simulink model "T_TypeInvPOb_07042020"  (R2018a)
settings: Solver=VariableStepDiscrete  StartTime=0.0  StopTime=0.4  MaxStep=1e-4  RelTol=1e-3  EnableMultiTasking=on
InitFcn:
  | Fs=10000;
  | Ts = 1/Fs; Vd = 400;
  | Vrate = 220; Irate = 25;
  | Rload = Vrate/Irate;
  | 
  | 
  | Lf = 0.423e-3+0.429e-3; Cf = 20e-6;
  | Rf = 0.01; Rc = 0.05;
  | 
  | C = 470e-6;
libraries: powerlib x28, powerlib_meascontrol x1
settings Model: Creator=Nguyen Linh  LastModifiedBy=ADMIN
settings SolverCC: ZeroCrossAlgorithm=Adaptive  AutoInsertRateTranBlk=on
settings DataIOCC: LimitDataPoints=on  SaveFormat=Array
settings OptimizationCC: LifeSpan=inf
settings DebuggingCC: MaxConsecutiveZCsMsg=none  SFUnexpectedBacktrackingDiag=warning  SFNoUnconditionalDefaultTransitionDiag=warning  SFExecutionAtInitializationDiag=none
settings HardwareCC: ProdBitPerPointer=32  ProdBitPerSizeT=32  ProdBitPerPtrDiffT=32  ProdLargestAtomicFloat=None  ProdIntDivRoundTo=Undefined  ProdEndianess=Unspecified  ProdWordSize=32  ProdHWDeviceType=32-bit Generic
settings ModelReferenceCC: PropagateSignalLabelsOutOfModel=off
settings CodeAppCC: StateflowObjectComments=on
settings GRTTargetCC: TargetLangStandard=C89/C90 (ANSI)  GeneratePreprocessorConditionals=Disable all
settings ConfigComp: CovMetricSettings=dw  CovHtmlReporting=on  CovSaveCumulativeToWorkspaceVar=on  CovSaveSingleToWorkspaceVar=on  CovExternalEMLEnable=off
settings SimscapeCC: SimscapeNormalizeSystem=off

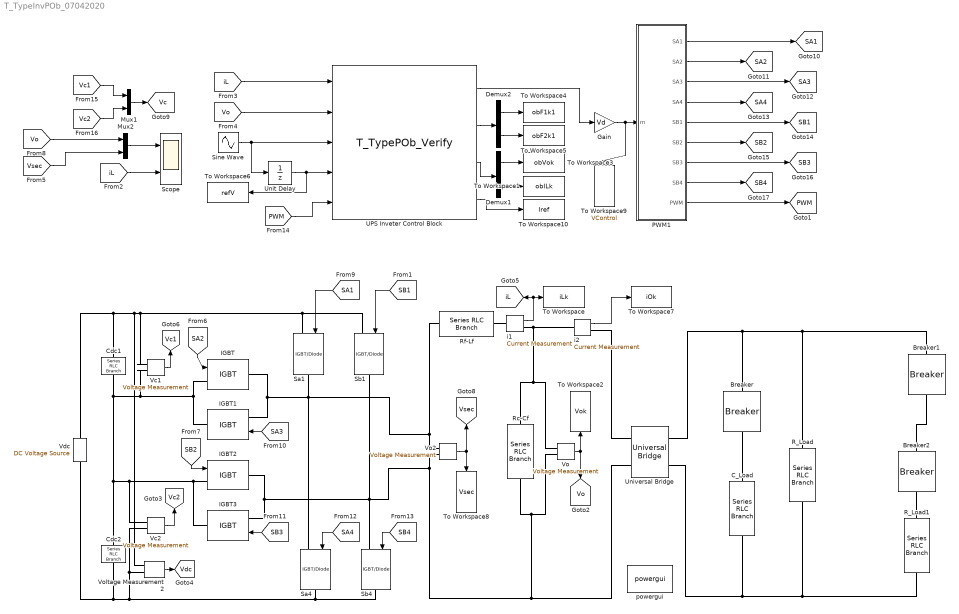
== system T_TypeInvPOb_07042020 ==
  Breaker : powerlib/Elements/Breaker  InitialState=1  SwitchingTimes=[0 0.25]  External=off  BreakerResistance=0.01  SnubberResistance=1e6  SnubberCapacitance=inf  Measurements=None  MoreParameters=on  NoBreakLoop=off
      settings: SourceProductName=Simscape Power Systems
  Breaker1 : powerlib/Elements/Breaker  InitialState=1  SwitchingTimes=[0 0.125]  External=off  BreakerResistance=0.01  SnubberResistance=1e6  SnubberCapacitance=inf  Measurements=None  MoreParameters=on  NoBreakLoop=off
      settings: SourceProductName=Simscape Power Systems
  Breaker2 : powerlib/Elements/Breaker  InitialState=0  SwitchingTimes=[0 0.185]  External=off  BreakerResistance=0.01  SnubberResistance=1e6  SnubberCapacitance=inf  Measurements=None  MoreParameters=on  NoBreakLoop=off
      settings: SourceProductName=Simscape Power Systems
  C_Load : powerlib/Elements/Series RLC Branch  LConnTagsString=__new0  RConnTagsString=__new0  BranchType=RC  Resistance=1  Inductance=1e-3  SetiL0=off  InitialCurrent=0  Capacitance=100e-6  Setx0=off  InitialVoltage=0  Measurements=None
  Cdc1 : powerlib/Elements/Series RLC Branch  LConnTagsString=__new0  RConnTagsString=__new0  BranchType=RC  Resistance=0.01  Inductance=0  SetiL0=off  InitialCurrent=0  Capacitance=C*2  Setx0=on  InitialVoltage=Vd/2  Measurements=Branch voltage and current
  Cdc2 : powerlib/Elements/Series RLC Branch  LConnTagsString=__new0  RConnTagsString=__new0  BranchType=RC  Resistance=0.01  Inductance=0  SetiL0=off  InitialCurrent=0  Capacitance=C*2  Setx0=on  InitialVoltage=Vd/2  Measurements=Branch voltage and current
  Demux1 : Demux  Outputs=2
  Demux2 : Demux  Outputs=2
  Gain : Gain  Gain=Vd
  IGBT{,1..3} (4 alike) : powerlib/Power Electronics/IGBT  Ron=0.001  Lon=0  Vf=1  Tf=1e-6  Tt=2e-6  IC=0  Rs=1e5  Cs=inf  Measurements=off
  Mux1 : Mux  Inputs=2
  Mux2 : Mux  Inputs=2
  PWM1 : Subsystem
  R_Load : powerlib/Elements/Series RLC Branch  LConnTagsString=__new0  RConnTagsString=__new0  BranchType=R  Resistance=100  Inductance=1e-3  SetiL0=off  InitialCurrent=0  Capacitance=1e-6  Setx0=off  InitialVoltage=0  Measurements=None
  R_Load1 : powerlib/Elements/Series RLC Branch  LConnTagsString=__new0  RConnTagsString=__new0  BranchType=R  Resistance=10  Inductance=1e-3  SetiL0=off  InitialCurrent=0  Capacitance=1e-6  Setx0=off  InitialVoltage=0  Measurements=None
  Rc-Cf : powerlib/Elements/Series RLC Branch  LConnTagsString=__new0  RConnTagsString=__new0  BranchType=RC  Resistance=Rc  Inductance=1e-3  SetiL0=off  InitialCurrent=0  Capacitance=Cf  Setx0=off  InitialVoltage=0  Measurements=None
  Rf-Lf : powerlib/Elements/Series RLC Branch  LConnTagsString=__new0  RConnTagsString=__new0  BranchType=RL  Resistance=Rf  Inductance=Lf  SetiL0=off  InitialCurrent=0  Capacitance=1e-6  Setx0=off  InitialVoltage=0  Measurements=None
  Sa1 : powerlib/Power Electronics/IGBT//Diode  Ron=1e-3  Rs=1e5  Cs=inf  Measurements=off
  Sa4 : powerlib/Power Electronics/IGBT//Diode  Ron=1e-3  Rs=1e5  Cs=inf  Measurements=off
  Sb1 : powerlib/Power Electronics/IGBT//Diode  Ron=1e-3  Rs=1e5  Cs=inf  Measurements=off
  Sb4 : powerlib/Power Electronics/IGBT//Diode  Ron=1e-3  Rs=1e5  Cs=inf  Measurements=off
  Scope : Scope  NumInputPorts=2
  Sine Wave : Sin  Amplitude=220*sqrt(2)  Frequency=2*pi*50  SampleTime=1/Fs
  To Workspace : ToWorkspace  VariableName=iLk  SaveFormat=Structure With Time  SampleTime=1e-6
  To Workspace1 : ToWorkspace  VariableName=obILk  SaveFormat=Structure With Time  SampleTime=1e-4
  To Workspace10 : ToWorkspace  VariableName=Iref  SaveFormat=Structure With Time  SampleTime=1e-4
  To Workspace2 : ToWorkspace  VariableName=Vok  SaveFormat=Structure With Time  SampleTime=1e-6
  To Workspace3 : ToWorkspace  VariableName=obVok  SaveFormat=Structure With Time  SampleTime=1e-4
  To Workspace4 : ToWorkspace  VariableName=obF1k1  SaveFormat=Structure With Time  SampleTime=1e-4
  To Workspace5 : ToWorkspace  VariableName=obF2k1  SaveFormat=Structure With Time  SampleTime=1e-4
  To Workspace6 : ToWorkspace  VariableName=refV  SaveFormat=Structure With Time  SampleTime=1e-4
  To Workspace7 : ToWorkspace  VariableName=iOk  SaveFormat=Structure With Time  SampleTime=5e-8
  To Workspace8 : ToWorkspace  VariableName=Vsec  SaveFormat=Structure With Time  SampleTime=1e-6
  To Workspace9 : ToWorkspace  VariableName=VControl  SaveFormat=Structure With Time  SampleTime=1e-6
  UPS Inveter Control Block : S-Function  InitFcn=try, set_param(gcb,'FunctionName','T_TypePOb_Verify'), end  FunctionName=T_TypePOb_Verify  SFunctionModules=T_TypePOb_Verify_wrapper  SFunctionDeploymentMode=off  EnableBusSupport=off  mask(S-Function Builder){}
      mask help: Simulink:masks:SFunctionBuilder_MD
      mask init:
      | val = [[.9  0.75 0.75 1 1 .9 .9 1]',[1 1 0.75 0.75 .9 .9 1 .9]'];try , sys = get_param(gcb,'SfunBuilderFcnName');if isempty(sys), sys = get_param(gcb,'FunctionName'); end,catch, sys = get_param(gcb,'FunctionName'); end
      settings: CopyFcn=set_param(gcbh,'LinkStatus','none')  PreSaveFcn=try, set_param(gcb,'FunctionName','T_TypePOb_Verify'), end  OpenFcn=sfunctionwizard(gcbh)
      mask Display: plot(val(:,1),val(:,2)),disp(sys), port_label('input',1,'iL'), port_label('input',2,'Vo'), port_label('input',3,'Vo_refk1'), port_label('input',4,'Vo_refk'), port_label('input',5,'PWM'), port_label('output',1,'D'), port_label('output',2,'obFk'), port_label('output',3,'obXk'), port_label('output',4,'Iref')
  Unit Delay : UnitDelay  SampleTime=1/Fs
  Universal Bridge : powerlib/Power Electronics/Universal Bridge  Arms=2  SnubberResistance=1e5  SnubberCapacitance=inf  Device=Diodes  Ron=1e-3  Lon=0  ForwardVoltages="[  0  0  ]"  ForwardVoltage=0  GTOparameters=[ 10e-6 , 20e-6 ]  IGBTparameters=[ 1e-6 , 2e-6 ]  Measurements=None  Measurements_2=None  converterType=Rectifier
  Vc1 : powerlib/Measurements/Voltage Measurement  PhasorSimulation=off  OutputType=Complex  PSBequivalent=0
  Vc2 : powerlib/Measurements/Voltage Measurement  PhasorSimulation=off  OutputType=Complex  PSBequivalent=0
  Vdc : powerlib/Electrical Sources/DC Voltage Source  Amplitude=Vd  Measurements=None
  Vo : powerlib/Measurements/Voltage Measurement  PhasorSimulation=off  OutputType=Complex  PSBequivalent=0
  Vo2 : powerlib/Measurements/Voltage Measurement  PhasorSimulation=off  OutputType=Complex  PSBequivalent=0
  Voltage Measurement2 : powerlib/Measurements/Voltage Measurement  PhasorSimulation=off  OutputType=Complex  PSBequivalent=0
  i1 : powerlib/Measurements/Current Measurement  PhasorSimulation=off  OutputType=Complex  PSBequivalent=0
  i2 : powerlib/Measurements/Current Measurement  PhasorSimulation=off  OutputType=Complex  PSBequivalent=0
  powergui : powerlib/powergui  Priority=1  SimulationMode=Discrete  SampleTime=5e-8  frequency=60  Iterations=50  frequencyindice=0  Pbase=100e6  ErrMax=1e-4  UnitsV=kV  UnitsW=MW  buscounter=0  FunctionMessages=off  echomessages=off  EnableUseOfTLC=off  CurrentSourceSwitches=off  DisableSnubberDevices=off  DisableRonSwitches=off  DisableVfSwitches=off  DisplayEquations=off  SolverType=Tustin/Backward Euler (TBE)  Interpol=off  ExternalGateDelay=off  methode=off  Ts=100  x0status=blocks  SPID=off  SwTol=0  HookPort=off  RestoreLinks=warning  ResistiveCurrentMeasurement=off  Frange=[0:2:500]  Ylog=off  Xlog=on  ShowGrid=off  save=off  variable=ZData  structure=Vok  ZoomFFT=on  StartTime=0.15  cycles=5  DisplayStyle=1  fundamental=50  FreqAxis=on  MaxFrequency=10000  frequencyindicesteady=1  RmsSteady=1  display=off
  tag scope: PWM=global, SA1=global, SA2=global, SA3=global, SA4=global, SB1=global, SB2=global, SB3=global, SB4=global, Vc1=global, Vc2=global, Vc=global, Vdc=global, Vo=global, Vsec=global, iL=global
  wires:
  i1/1 -> To Workspace/1, [iL]
  Vo/1 -> [Vo], To Workspace2/1
  Vo2/1 -> To Workspace8/1, [Vsec]
  Voltage Measurement2/1 -> [Vdc]
  [SB4] -> Sb4/1
  [SA1] -> Sa1/1
  [SA2] -> IGBT/1
  [SB2] -> IGBT2/1
  [SA3] -> IGBT1/1
  [SB1] -> Sb1/1
  [SB3] -> IGBT3/1
  [SA4] -> Sa4/1
  Vc2/1 -> [Vc2]
  Vc1/1 -> [Vc1]
  [Vc1] -> Mux1/1
  [PWM] -> UPS Inveter Control Block/5
  UPS Inveter Control Block/1 -> Gain/1
  PWM1/7(SB3) -> [SB3]
  [Vc2] -> Mux1/2
  Gain/1 -> To Workspace9/1, PWM1/1(m)
  PWM1/5(SB1) -> [SB1]
  PWM1/1(SA1) -> [SA1]
  Demux2/1 -> To Workspace4/1
  PWM1/4(SA4) -> [SA4]
  PWM1/8(SB4) -> [SB4]
  PWM1/2(SA2) -> [SA2]
  PWM1/9(PWM) -> [PWM]
  PWM1/6(SB2) -> [SB2]
  UPS Inveter Control Block/2 -> Demux2/1
  PWM1/3(SA3) -> [SA3]
  Sine Wave/1 -> UPS Inveter Control Block/3, Unit Delay/1
  UPS Inveter Control Block/3 -> Demux1/1
  [iL] -> UPS Inveter Control Block/1
  Demux2/2 -> To Workspace5/1
  Demux1/1 -> To Workspace3/1
  Mux1/1 -> [Vc]
  Demux1/2 -> To Workspace1/1
  Unit Delay/1 -> UPS Inveter Control Block/4, To Workspace6/1
  [Vo] -> UPS Inveter Control Block/2
  UPS Inveter Control Block/4 -> To Workspace10/1
  Mux2/1 -> Scope/1
  [Vo] -> Mux2/1
  [Vsec] -> Mux2/2
  [iL] -> Scope/2
  i2/1 -> To Workspace7/1
  connections:
  Sb4/LConn1 -- IGBT3/LConn1 -- IGBT2/RConn1 -- Sb1/RConn1 -- Vo/LConn2 -- Rc-Cf/RConn1 -- Universal Bridge/LConn2 -- Vo2/LConn2
  IGBT/RConn1 -- Rf-Lf/LConn1 -- Vo2/LConn1 -- Sa4/LConn1 -- Sa1/RConn1 -- IGBT1/LConn1
  i1/RConn1 -- i2/LConn1 -- Vo/LConn1 -- Rc-Cf/LConn1
  Rf-Lf/RConn1 -- i1/LConn1
  IGBT/LConn1 -- Cdc1/RConn1 -- Vc2/LConn1 -- IGBT3/RConn1 -- IGBT2/LConn1 -- Cdc2/LConn1 -- Vc1/LConn2 -- IGBT1/RConn1
  Sb4/RConn1 -- Vdc/LConn1 -- Cdc2/RConn1 -- Voltage Measurement2/LConn2 -- Vc2/LConn2 -- Sa4/RConn1
  Sa1/LConn1 -- Vdc/RConn1 -- Cdc1/LConn1 -- Voltage Measurement2/LConn1 -- Vc1/LConn1 -- Sb1/LConn1
  Universal Bridge/RConn2 -- R_Load/RConn1 -- R_Load1/RConn1 -- C_Load/RConn1
  R_Load/LConn1 -- Universal Bridge/RConn1 -- Breaker/LConn1 -- Breaker1/LConn1
  Universal Bridge/LConn1 -- i2/RConn1
  Breaker/RConn1 -- C_Load/LConn1
  Breaker2/RConn1 -- R_Load1/LConn1
  Breaker1/RConn1 -- Breaker2/LConn1

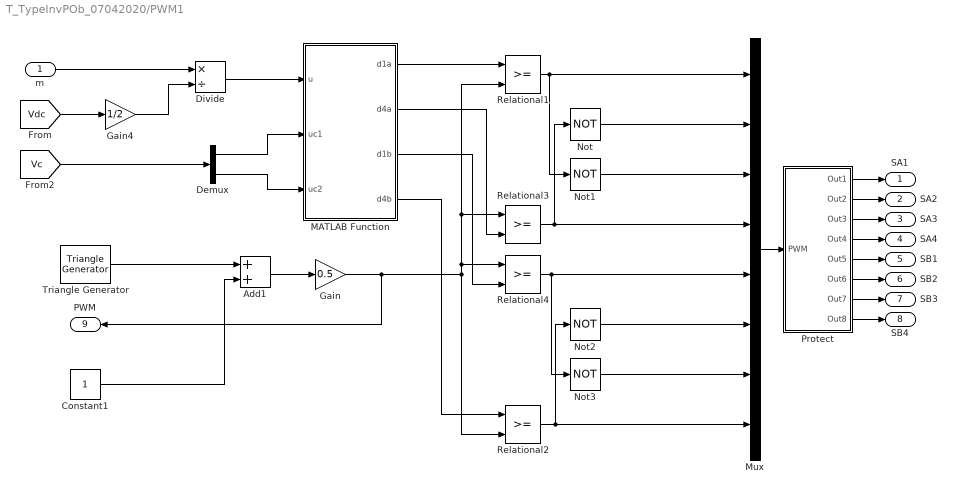
== system T_TypeInvPOb_07042020/PWM1 ==
  m : Inport
  Add1 : Sum
  Constant1 : Constant
  Demux : Demux  Outputs=2
  Divide : Product  Inputs=*/
  Gain : Gain  Gain=0.5
  Gain4 : Gain  Gain=1/2
  MATLAB Function : MATLAB Function  TreatAsAtomicUnit=on
  Mux : Mux  Inputs=8
  Not{,1..3} (4 alike) : Logic  Operator=NOT  AllPortsSameDT=off  OutDataTypeStr=boolean
  Protect : Subsystem
  Relational{1..4} (4 alike) : RelationalOperator  OutDataTypeStr=boolean  RndMeth=Nearest  InputSameDT=on
  Triangle Generator : powerlib_meascontrol/Pulse & Signal Generators/Triangle Generator  Freq=Fs/2  Phase=0  Ts=0
  SA1 : Outport
  SA2 : Outport  Port=2
  SA3 : Outport  Port=3
  SA4 : Outport  Port=4
  SB1 : Outport  Port=5
  SB2 : Outport  Port=6
  SB3 : Outport  Port=7
  SB4 : Outport  Port=8
  PWM : Outport  Port=9
  wires:
  Add1/1 -> Gain/1
  Constant1/1 -> Add1/2
  Gain/1 -> PWM/1, Relational4/1, Relational1/2, Relational3/1, Relational2/2
  [Vdc] -> Gain4/1
  Gain4/1 -> Divide/2
  m/1 -> Divide/1
  Divide/1 -> MATLAB Function/1(u)
  MATLAB Function/1(d1a) -> Relational1/1
  MATLAB Function/2(d4a) -> Relational3/2
  MATLAB Function/3(d1b) -> Relational4/2
  MATLAB Function/4(d4b) -> Relational2/1
  Demux/1 -> MATLAB Function/2(uc1)
  Demux/2 -> MATLAB Function/3(uc2)
  Relational1/1 -> Mux/1, Not1/1
  Not/1 -> Mux/2
  Relational3/1 -> Mux/4, Not/1
  Relational4/1 -> Mux/5, Not3/1
  Not3/1 -> Mux/7
  Relational2/1 -> Mux/8, Not2/1
  Triangle Generator/1 -> Add1/1
  [Vc] -> Demux/1
  Mux/1 -> Protect/1(PWM)
  Protect/1(Out1) -> SA1/1
  Protect/2(Out2) -> SA2/1
  Protect/3(Out3) -> SA3/1
  Protect/4(Out4) -> SA4/1
  Protect/5(Out5) -> SB1/1
  Protect/6(Out6) -> SB2/1
  Protect/7(Out7) -> SB3/1
  Protect/8(Out8) -> SB4/1
  Not1/1 -> Mux/3
  Not2/1 -> Mux/6

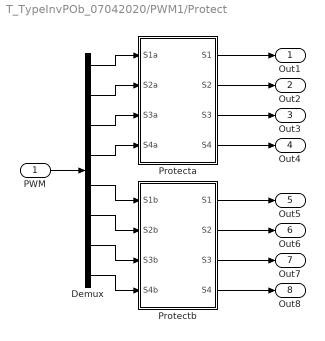
== system T_TypeInvPOb_07042020/PWM1/Protect ==
  PWM : Inport
  Demux : Demux  Outputs=8
  Protecta : Subsystem
  Protectb : Subsystem
  Out1 : Outport
  Out2 : Outport  Port=2
  Out3 : Outport  Port=3
  Out4 : Outport  Port=4
  Out5 : Outport  Port=5
  Out6 : Outport  Port=6
  Out7 : Outport  Port=7
  Out8 : Outport  Port=8
  wires:
  Protectb/2(S2) -> Out6/1
  Demux/3 -> Protecta/3(S3a)
  Demux/4 -> Protecta/4(S4a)
  Demux/2 -> Protecta/2(S2a)
  Protectb/3(S3) -> Out7/1
  Protectb/4(S4) -> Out8/1
  Demux/1 -> Protecta/1(S1a)
  Protectb/1(S1) -> Out5/1
  Protecta/4(S4) -> Out4/1
  Protecta/3(S3) -> Out3/1
  Protecta/2(S2) -> Out2/1
  Protecta/1(S1) -> Out1/1
  Demux/5 -> Protectb/1(S1b)
  Demux/6 -> Protectb/2(S2b)
  Demux/7 -> Protectb/3(S3b)
  Demux/8 -> Protectb/4(S4b)
  PWM/1 -> Demux/1

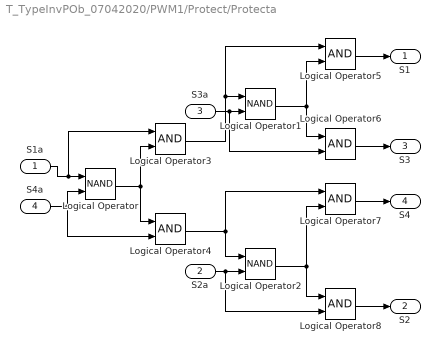
== system T_TypeInvPOb_07042020/PWM1/Protect/Protecta ==
  S1a : Inport
  S2a : Inport  Port=2
  S3a : Inport  Port=3
  S4a : Inport  Port=4
  Logical Operator : Logic  Operator=NAND  AllPortsSameDT=off  OutDataTypeStr=boolean
  Logical Operator1 : Logic  Operator=NAND  AllPortsSameDT=off  OutDataTypeStr=boolean
  Logical Operator2 : Logic  Operator=NAND  AllPortsSameDT=off  OutDataTypeStr=boolean
  Logical Operator{3..8} (6 alike) : Logic  AllPortsSameDT=off  OutDataTypeStr=boolean
  S1 : Outport
  S2 : Outport  Port=2
  S3 : Outport  Port=3
  S4 : Outport  Port=4
  wires:
  Logical Operator5/1 -> S1/1
  Logical Operator7/1 -> S4/1
  Logical Operator8/1 -> S2/1
  Logical Operator/1 -> Logical Operator4/1, Logical Operator3/2
  Logical Operator6/1 -> S3/1
  Logical Operator4/1 -> Logical Operator7/1, Logical Operator2/1
  Logical Operator1/1 -> Logical Operator5/2, Logical Operator6/1
  Logical Operator3/1 -> Logical Operator5/1, Logical Operator1/1
  Logical Operator2/1 -> Logical Operator7/2, Logical Operator8/1
  S1a/1 -> Logical Operator3/1, Logical Operator/1
  S4a/1 -> Logical Operator4/2, Logical Operator/2
  S3a/1 -> Logical Operator6/2, Logical Operator1/2
  S2a/1 -> Logical Operator8/2, Logical Operator2/2

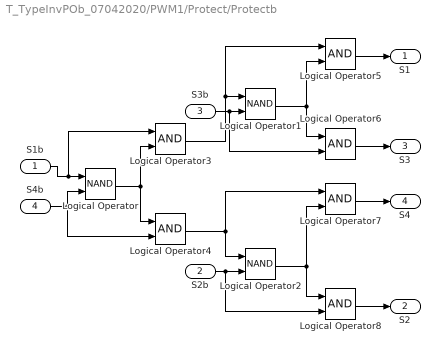
== system T_TypeInvPOb_07042020/PWM1/Protect/Protectb ==
  S1b : Inport
  S2b : Inport  Port=2
  S3b : Inport  Port=3
  S4b : Inport  Port=4
  Logical Operator : Logic  Operator=NAND  AllPortsSameDT=off  OutDataTypeStr=boolean
  Logical Operator1 : Logic  Operator=NAND  AllPortsSameDT=off  OutDataTypeStr=boolean
  Logical Operator2 : Logic  Operator=NAND  AllPortsSameDT=off  OutDataTypeStr=boolean
  Logical Operator{3..8} (6 alike) : Logic  AllPortsSameDT=off  OutDataTypeStr=boolean
  S1 : Outport
  S2 : Outport  Port=2
  S3 : Outport  Port=3
  S4 : Outport  Port=4
  wires:
  S2b/1 -> Logical Operator2/2, Logical Operator8/2
  S3b/1 -> Logical Operator1/2, Logical Operator6/2
  S4b/1 -> Logical Operator/2, Logical Operator4/2
  S1b/1 -> Logical Operator/1, Logical Operator3/1
  Logical Operator2/1 -> Logical Operator8/1, Logical Operator7/2
  Logical Operator3/1 -> Logical Operator1/1, Logical Operator5/1
  Logical Operator1/1 -> Logical Operator6/1, Logical Operator5/2
  Logical Operator4/1 -> Logical Operator2/1, Logical Operator7/1
  Logical Operator6/1 -> S3/1
  Logical Operator/1 -> Logical Operator3/2, Logical Operator4/1
  Logical Operator8/1 -> S2/1
  Logical Operator7/1 -> S4/1
  Logical Operator5/1 -> S1/1

== matlab function T_TypeInvPOb_07042020/PWM1/MATLAB Function ==
  data: u input; d1a output; d4a output; d1b output; d4b output; uc1 input; uc2 input
function [d1a,d4a,d1b,d4b] = Duty(u,uc1,uc2)
%#codegen
%a
if (uc1 <= uc2) 
    d1a = u - 1;
else 
    d1a = u;
end
if (uc1 >= uc2);
    d4a = u + 2;
else 
    d4a = u + 1;
end

%b
if (uc1 >= uc2);
    d1b = u + 1;
else
    d1b = u + 2;
end
if (uc1 <= uc2) 
    d4b = u;
else
    d4b = u - 1;
end
end
